simulink model "qdqd_robot"  (R2022b)
settings: Solver=FixedStepAuto  StartTime=0.0  StopTime=inf  FixedStep=0.01  RelTol=1e-3  EnableMultiTasking=on
model workspace: external: MATLAB File C:\Users\Tin\Desktop\tailieuhoc\TT Robotics\task2\robot_DataFile2.m (data not in the file)
libraries: arduinolib x3
settings Model: ExtModeTrigDuration=2  Creator=Tin  LastModifiedBy=Admin
settings OptimizationCC: EnhancedBackFolding=on  PassReuseOutputArgsAs=Individual arguments  ZeroExternalMemoryAtStartup=off  ZeroInternalMemoryAtStartup=off  MaxStackSize=64  OptimizeBlockOrder=speed  DifferentSizesBufferReuse=on  OptimizationCustomize=off  EfficientTunableParamExpr=on
settings DebuggingCC: ParameterTunabilityLossMsg=error
settings HardwareCC: ProdBitPerInt=16  ProdBitPerPointer=16  ProdBitPerSizeT=16  ProdBitPerPtrDiffT=16  ProdLargestAtomicFloat=None  ProdWordSize=8  ProdHWDeviceType=Atmel->AVR
settings SFSimCC: MATLABDynamicMemAlloc=off
settings RTWCC: Description=Embedded Coder  SystemTargetFile=ert.tlc  HardwareBoard=Arduino Uno  TLCOptions=-aInlineSetEventsForThisBaseRateFcn=TLC_FALSE -aSuppressMultiTaskScheduler=TLC_FALSE -aRateBasedStepFcn=1  TemplateMakefile=ert_default_tmf  Toolchain=Arduino AVR  BuildConfiguration=Faster Runs
settings CodeAppCC: ForceParamTrailComments=on  IgnoreCustomStorageClasses=off  OperatorAnnotations=on  SimulinkDataObjDesc=on  SFDataObjDesc=on  InsertBlockDesc=on
settings ERTTargetCC: SupportContinuousTime=on  SupportVariableSizeSignals=on  ExtModeTransport=3  ExtModeStaticAlloc=on  ExtModeAutomaticAllocSize=off  ExtModeStaticAllocSize=250  ExtModeMexFile=ext_xcp  ExtModeIntrfLevel=Level2 - Open

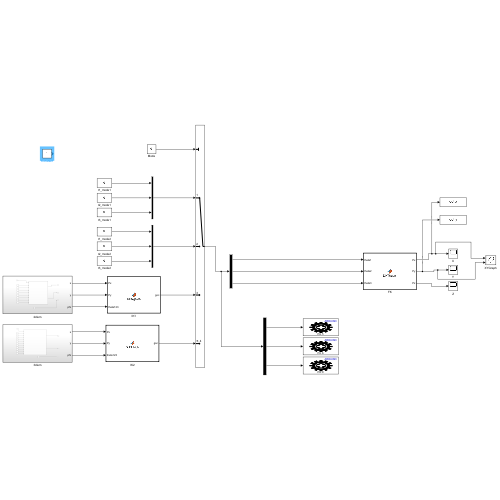
[thumbnail: Simulink's stored preview of the top-level diagram]
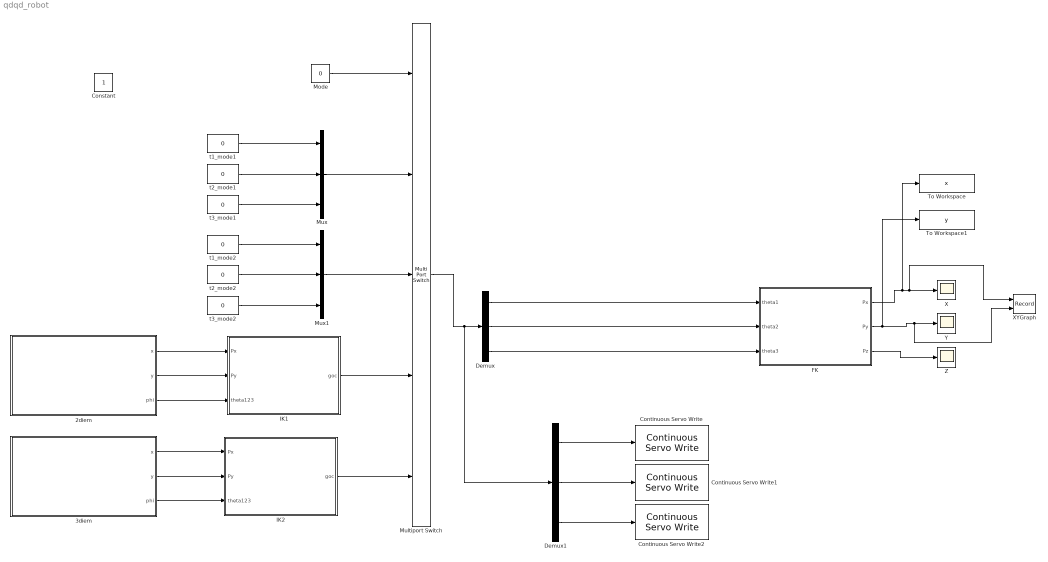
== system qdqd_robot ==
  2diem : Subsystem
  3diem : Subsystem
  Constant : Constant
  Continuous Servo Write : arduinolib/Continuous Servo Write  pinNumber=5  ServoIndex=0  blockPlatform=ARDUINO
  Continuous Servo Write1 : arduinolib/Continuous Servo Write  pinNumber=6  ServoIndex=1  blockPlatform=ARDUINO
  Continuous Servo Write2 : arduinolib/Continuous Servo Write  pinNumber=9  ServoIndex=2  blockPlatform=ARDUINO
  Demux : Demux  Outputs=3
  Demux1 : Demux  Outputs=3
  FK : MATLAB Function  TreatAsAtomicUnit=on
  IK1 : MATLAB Function  TreatAsAtomicUnit=on
  IK2 : MATLAB Function  TreatAsAtomicUnit=on
  Mode : Constant  Value=0
  Multiport Switch : MultiPortSwitch  Inputs=4  DiagnosticForDefault=None  SaturateOnIntegerOverflow=off  InputSameDT=off
  Mux : Mux  Inputs=3
  Mux1 : Mux  Inputs=3
  To Workspace : ToWorkspace  VariableName=x  SampleTime=-1
      settings: Save2DSignal=2-D array (concatenate along first dimension)
  To Workspace1 : ToWorkspace  VariableName=y  SampleTime=-1
      settings: Save2DSignal=2-D array (concatenate along first dimension)
  X : Scope
  XYGraph : Record  FileSettingsInternal="{\"entries\":[{\"content\":{\"excelSettings\":{\"content\":{},\"type\":\"Streamout.ExcelSettings\"}},\"type\":\"Streamout.FileSettingStorage\",\"uuid\":\"40183822-63cf-417b-8100-ac02f2e21893\"}],\"packageUris\":[\"http://schema.mathworks.com/mf0/streamout_blocks/R2020a\"],\"version\":\"1.0\"}"  Layout=[1 1]  SignalsInternal="{\"entries\":[{\"content\":{\"signals\":[{\"content\":{\"blockPath\":[\"qdqd_robot/XYGraph\"],\"channel\":[],\"dimensions\":[1],\"domain\":\"qdqd_robot/XYGraph\",\"lineColor\":\"#ff6929\",\"plots\":[],\"port\":1,\"sid\":[],\"signalID\":8,\"signalName\":\"FK:1\"},\"type\":\"RecordBlkView.Signal\",\"uuid\":\"95a28990-beca-47bf-8945-fb8e86b36b02\"},{\"content\":{\"blockPath\":[\"qdqd_robot/XYGraph\"],\"channel\":[],\"dimensions\":[1],\"domain\":\"qdqd_robot/XYGraph\",\"lineColor\":\"#b746ff\",\"plots\":[],\"port\":2,\"sid\":[],\"signalID\":11,\"signalName\":\"FK:2\"},\"type\":\"RecordBlkView.Signal\",\"uuid\":\"91a18261-c3c3-431b-839b-3cfd5142652e\"}]},\"type\":\"RecordBlkView.InputSignals\",\"uuid\":\"2a646766-b014-4e68-8631-8a488f9ec856\"}],\"packageUris\":[\"http://schema.mathworks.com/mf0/streamout_blocks/R2020a\"],\"version\":\"1.0\"}"  VisualizationBindings="{\"xyplotplugin\":{\"info\":[{\"series\":[],\"subplotID\":1}]}}"  CompatibilityTag=XY
  Y : Scope
  Z : Scope
  t1_mode1 : Constant  Value=0
  t1_mode2 : Constant  Value=0
  t2_mode1 : Constant  Value=0
  t2_mode2 : Constant  Value=0
  t3_mode1 : Constant  Value=0
  t3_mode2 : Constant  Value=0
  wires:
  2diem/3(phi) -> IK1/3(theta123)
  2diem/2(y) -> IK1/2(Py)
  3diem/3(phi) -> IK2/3(theta123)
  t2_mode1/1 -> Mux/2
  t3_mode1/1 -> Mux/3
  Mux/1 -> Multiport Switch/2
  Multiport Switch/1 -> Demux1/1, Demux/1
  t1_mode1/1 -> Mux/1
  3diem/2(y) -> IK2/2(Py)
  3diem/1(x) -> IK2/1(Px)
  FK/1(Px) -> To Workspace/1, XYGraph/1, X/1
  FK/2(Py) -> To Workspace1/1, XYGraph/2, Y/1
  FK/3(Pz) -> Z/1
  2diem/1(x) -> IK1/1(Px)
  Mode/1 -> Multiport Switch/1
  IK2/1(goc) -> Multiport Switch/5
  IK1/1(goc) -> Multiport Switch/4
  t1_mode2/1 -> Mux1/1
  Mux1/1 -> Multiport Switch/3
  t3_mode2/1 -> Mux1/3
  t2_mode2/1 -> Mux1/2
  Demux/1 -> FK/1(theta1)
  Demux/2 -> FK/2(theta2)
  Demux/3 -> FK/3(theta3)
  Demux1/1 -> Continuous Servo Write/1
  Demux1/2 -> Continuous Servo Write1/1
  Demux1/3 -> Continuous Servo Write2/1

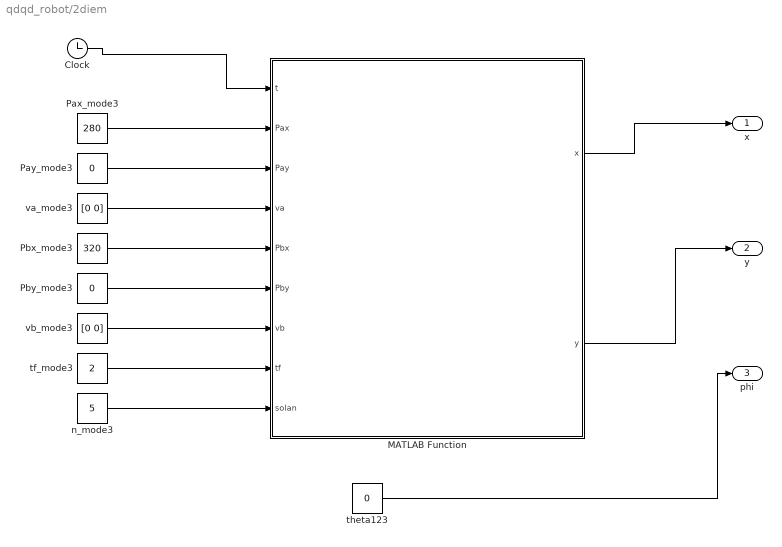
== system qdqd_robot/2diem ==
  Clock : Clock
  MATLAB Function : MATLAB Function  TreatAsAtomicUnit=on
  Pax_mode3 : Constant  Value=280
  Pay_mode3 : Constant  Value=0
  Pbx_mode3 : Constant  Value=320
  Pby_mode3 : Constant  Value=0
  n_mode3 : Constant  Value=5
  tf_mode3 : Constant  Value=2
  theta123 : Constant  Value=0
  va_mode3 : Constant  Value=[0 0]
  vb_mode3 : Constant  Value=[0 0]
  x : Outport
  y : Outport  Port=2
  phi : Outport  Port=3
  wires:
  Pbx_mode3/1 -> MATLAB Function/5(Pbx)
  Pax_mode3/1 -> MATLAB Function/2(Pax)
  Pby_mode3/1 -> MATLAB Function/6(Pby)
  Clock/1 -> MATLAB Function/1(t)
  tf_mode3/1 -> MATLAB Function/8(tf)
  n_mode3/1 -> MATLAB Function/9(solan)
  vb_mode3/1 -> MATLAB Function/7(vb)
  va_mode3/1 -> MATLAB Function/4(va)
  Pay_mode3/1 -> MATLAB Function/3(Pay)
  MATLAB Function/1(x) -> x/1
  theta123/1 -> phi/1
  MATLAB Function/2(y) -> y/1

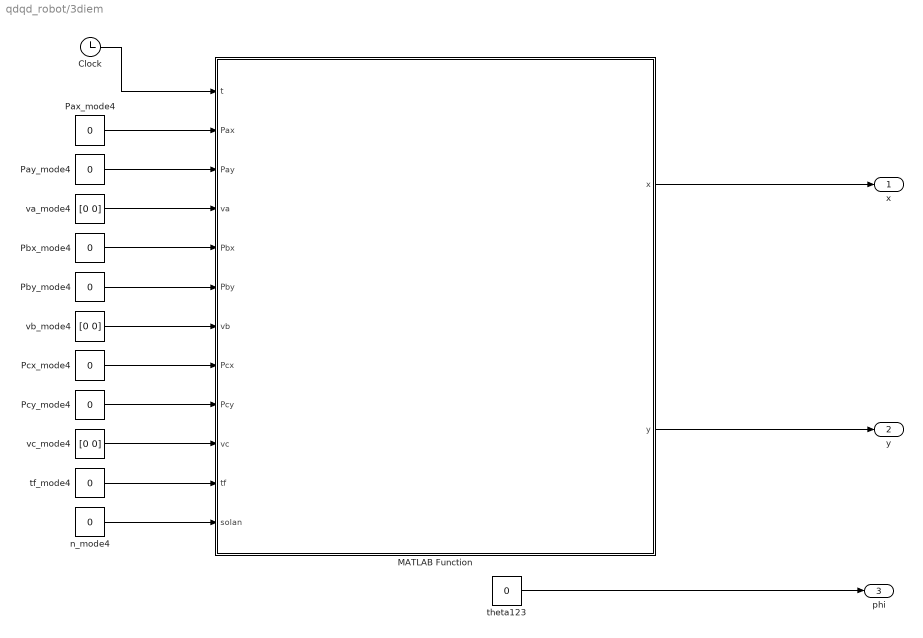
== system qdqd_robot/3diem ==
  Clock : Clock
      settings: Decimation=30
  MATLAB Function : MATLAB Function  TreatAsAtomicUnit=on
  Pax_mode4 : Constant  Value=0
  Pay_mode4 : Constant  Value=0
  Pbx_mode4 : Constant  Value=0
  Pby_mode4 : Constant  Value=0
  Pcx_mode4 : Constant  Value=0
  Pcy_mode4 : Constant  Value=0
  n_mode4 : Constant  Value=0
  tf_mode4 : Constant  Value=0
  theta123 : Constant  Value=0
  va_mode4 : Constant  Value=[0 0]
  vb_mode4 : Constant  Value=[0 0]
  vc_mode4 : Constant  Value=[0 0]
  x : Outport
  y : Outport  Port=2
  phi : Outport  Port=3
  wires:
  theta123/1 -> phi/1
  Pcx_mode4/1 -> MATLAB Function/8(Pcx)
  Pcy_mode4/1 -> MATLAB Function/9(Pcy)
  Pbx_mode4/1 -> MATLAB Function/5(Pbx)
  vc_mode4/1 -> MATLAB Function/10(vc)
  tf_mode4/1 -> MATLAB Function/11(tf)
  Pax_mode4/1 -> MATLAB Function/2(Pax)
  va_mode4/1 -> MATLAB Function/4(va)
  Clock/1 -> MATLAB Function/1(t)
  Pby_mode4/1 -> MATLAB Function/6(Pby)
  Pay_mode4/1 -> MATLAB Function/3(Pay)
  vb_mode4/1 -> MATLAB Function/7(vb)
  n_mode4/1 -> MATLAB Function/12(solan)
  MATLAB Function/1(x) -> x/1
  MATLAB Function/2(y) -> y/1

== matlab function qdqd_robot/IK1 ==
  data: Px input; goc output; Py input; theta123 input
function goc  = DHNghich(Px, Py, theta123)
     l0 = 80;
     l1 = 99.98;
     l2 = 95.14;
     l3 = 80;
     d1 = 122.4;
     d2 = 22.4;
     d3 = 18.85;

     % Tinh theta1 
     A = Px - l0 - l3*cosd(theta123);
     B = Py - l3*sind(theta123);
     a = 2*A*l1;
     b = 2*B*l1;
     d = A^2 + B^2 + l1^2 - l2^2;
     anpha = atan2d(a/sqrt(a^2+b^2), b/sqrt(a^2+b^2));
     s1 = d/sqrt(a^2+b^2);
     if(abs(s1 - 1) <= 0.0001)
            if(s1 > 0)
                 s1 = 1;
            else s1 = -1;
            end
     end
     c1 = sqrt(1 - s1^2);
     theta1 = atan2d(s1, c1) - anpha;
     % Tinh theta2
     s2 = (Py - l3*sind(theta123) - l1*sind(theta1)) / l2;
     c2 = (Px - l0 - l1*cosd(theta1) - l3*cosd(theta123))/l2;
     theta2 = atan2d(s2,c2) - theta1;
     % Tinh theta3
    theta3 = theta123 - theta1 - theta2;
    goc = [theta1; theta2; theta3];
end

== matlab function qdqd_robot/2diem/MATLAB Function ==
  data: x output; t input; y output; Pax input; Pay input; va input; Pbx input; Pby input; vb input; tf input; solan input
function [x, y] = QHQD2D(t, Pax, Pay, va, Pbx, Pby, vb, tf, solan)

    function [x, y] = TrajectoryPlanning(t, P0, v0, Pf, vf, tf, t0)
        a10 = P0(1);
        a20 = P0(2);
        a11 = v0(1);
        a21 = v0(2);  
    
        a12 = 3 / tf^2 * (Pf(1) - P0(1)) - 2 / tf * v0(1) - 1 / tf * vf(1);
        a22 = 3 / tf^2 * (Pf(2) - P0(2)) - 2 / tf * v0(2) - 1 / tf * vf(2);
        a13 = -2 / tf^3 * (Pf(1) - P0(1)) + 1 / tf^2 * (vf(1) + v0(1));
        a23 = -2 / tf^3 * (Pf(2) - P0(2)) + 1 / tf^2 * (vf(2) + v0(2));
    
        x = a10 + a11 *(t - t0) + a12 * (t - t0)^2 + a13*(t - t0)^3;
        y = a20 + a21 *(t - t0) + a22 * (t - t0)^2 + a23*(t - t0)^3;
    end

    chuky = tf*2;
    i = fix(t/chuky);
    Pa = [Pax Pay];
    Pb = [Pbx Pby];
    if(t <= (tf + chuky*i))
        [x, y] = TrajectoryPlanning(t, Pa, va, Pb, vb, tf, 0 + chuky * i);
    else
        [x, y] = TrajectoryPlanning(t, Pa, va, Pb, vb, tf, tf + chuky * i);
    end
    if(t > chuky*solan)
         x = Pax;
         y = Pay;
    end
end

== matlab function qdqd_robot/3diem/MATLAB Function ==
  data: x output; t input; y output; Pax input; Pay input; va input; Pbx input; Pby input; vb input; Pcx input; Pcy input; vc input; tf input; solan input
function [x, y] = QHQD3D(t, Pax, Pay, va, Pbx, Pby, vb, Pcx, Pcy, vc, tf, solan) 
    function [x, y, z] = TrajectoryPlanning(t, P0, v0, Pf, vf, tf, t0)
        a10 = P0(1);
        a20 = P0(2);
        a11 = v0(1);
        a21 = v0(2);  
    
        a12 = 3 / tf^2 * (Pf(1) - P0(1)) - 2 / tf * v0(1) - 1 / tf * vf(1);
        a22 = 3 / tf^2 * (Pf(2) - P0(2)) - 2 / tf * v0(2) - 1 / tf * vf(2);
        a13 = -2 / tf^3 * (Pf(1) - P0(1)) + 1 / tf^2 * (vf(1) + v0(1));
        a23 = -2 / tf^3 * (Pf(2) - P0(2)) + 1 / tf^2 * (vf(2) + v0(2));
    
        x = a10 + a11 *(t - t0) + a12 * (t - t0)^2 + a13*(t - t0)^3;
        y = a20 + a21 *(t - t0) + a22 * (t - t0)^2 + a23*(t - t0)^3;
        z = 0;
    end
    chuky = tf*3;
    i = fix(t/chuky);
    Pa = [Pax Pay];
    Pb = [Pbx Pby];
    Pc = [Pcx Pcy];
    if(t <= (tf + chuky*i))
        [x, y] = TrajectoryPlanning(t, Pa, va, Pb, vb, tf, tf*0 + chuky * i);
    elseif(t <= (tf*2 + chuky*i))
        [x, y] = TrajectoryPlanning(t, Pb, vb, Pc, vc, tf, tf*1 + chuky * i);
    else
        [x, y] = TrajectoryPlanning(t, Pc, vc, Pa, va, tf, tf*2 + chuky * i);
    end
    if(t > chuky*solan)
         x = Pax;
         y = Pay;
    end
end

== matlab function qdqd_robot/IK2 ==
  data: Px input; goc output; Py input; theta123 input
function goc  = DHNghich(Px, Py, theta123)
    l0 = 80;
     l1 = 99.98;
     l2 = 95.14;
     l3 = 80;
     d1 = 122.4;
     d2 = 22.4;
     d3 = 18.85;

     % Tinh theta1 
     A = Px - l0 - l3*cosd(theta123);
     B = Py - l3*sind(theta123);
     a = 2*A*l1;
     b = 2*B*l1;
     d = A^2 + B^2 + l1^2 - l2^2;
     anpha = atan2d(a/sqrt(a^2+b^2), b/sqrt(a^2+b^2));
     s1 = d/sqrt(a^2+b^2);
     if(abs(s1 - 1) <= 0.0001)
            if(s1 > 0)
                 s1 = 1;
            else s1 = -1;
            end
     end
     c1 = sqrt(1 - s1^2);
     theta1 = atan2d(s1, -c1) - anpha;
     % Tinh theta2
     s2 = (Py - l3*sind(theta123) - l1*sind(theta1)) / l2;
     c2 = (Px - l0 - l1*cosd(theta1) - l3*cosd(theta123))/l2;
     theta2 = atan2d(s2,c2) - theta1;
     % Tinh theta3
    theta3 = theta123 - theta1 - theta2;
    goc = [theta1; theta2; theta3];
end

== matlab function qdqd_robot/FK ==
  data: theta1 input; Px output; theta2 input; theta3 input; Py output; Pz output
function [Px, Py, Pz] = DHThuan(theta1, theta2, theta3)
    l1 = 100;
    l2 = 250;
    l3 = 250;
    l4 = 150;
    d1 = 30;
    d2 = 30;
    d3 = 30;
    l0 = 150;

    theta123= 0;

    Px = l1 + l2*cosd(theta1) + l3*cosd(theta1 + theta2) + l4*cosd(theta123);
    Py = l2*sind(theta1) + l3*sind(theta1 + theta2) + l4*sind(theta123);
    Pz = l0 + d1 + d2 + d3;
end
